simulink model "state_feedback"  (R2016b)
settings: Solver=ode45  StartTime=0.0  StopTime=10.0  RelTol=1e-3
values from neighbouring files (symbols this model uses):
  C = [1 0 0 0 0;0 0 1 0 0]    [cee_MACRO.m]
  D = [0 0 0 0 0]'    [cee_MACRO.m]
  K = lqr(A, B, Qr, Rr)    [cee_MACRO.m]
  x0c = deg2rad(x0c_graus)'    [cee_MACRO.m]
undefined symbols (not defined in the file or in its folder): A, B
settings Model: Creator=jmgri  LastModifiedBy=jmgri
settings OptimizationCC: LifeSpan=inf
settings DebuggingCC: SFExecutionAtInitializationDiag=none
settings HardwareCC: ProdBitPerSizeT=32  ProdBitPerPtrDiffT=32  ProdWordSize=32  ProdHWDeviceType=Specified

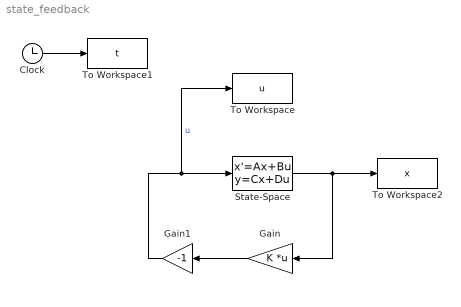
== system state_feedback ==
  Clock : Clock
  Gain : Gain  Gain=K  Multiplication=Matrix(K*u)
  Gain1 : Gain  Gain=-1
  State-Space : StateSpace  A=A  B=B  C=C  D=D  X0=x0c
  To Workspace : ToWorkspace  VariableName=u  SampleTime=-1
  To Workspace1 : ToWorkspace  VariableName=t  SampleTime=-1
  To Workspace2 : ToWorkspace  VariableName=x  SampleTime=-1
  wires:
  Gain/1 -> Gain1/1
  Gain1/1 -> To Workspace/1, State-Space/1  "u"
  State-Space/1 -> To Workspace2/1, Gain/1
  Clock/1 -> To Workspace1/1
